simulink model "proj_sim"  (R2024b)
settings: Solver=VariableStepAuto  StartTime=0.0  StopTime=inf  RelTol=1e-3
values from neighbouring files (symbols this model uses):
  gravitation = 9.82    [load_vars.m]
  Weight = scaler * (380 + 72.2)    (= 50.01332)    [load_vars.m]
undefined symbols (not defined in the file or in its folder): battery_voltage, current_limiting_resistor, max_current, Weight_of_tt
libraries: fl_lib x16, nesl_utility x9, sdl_lib x3, ee_lib x1, slpidlib x1, simulink_extras x1, simulink x1
(part 2 of 2)

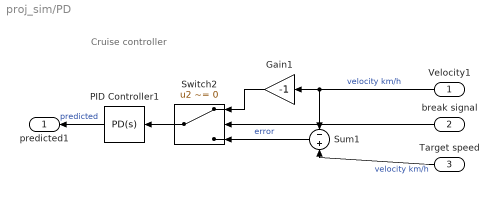
== system proj_sim/PD ==
  note: Cruise controller
  Velocity1 : Inport
  break signal : Inport  Port=2
  Target speed : Inport  Port=3
  Gain1 : Gain  Gain=-1
  PID Controller1 : slpidlib/PID Controller  Controller=PD  Form=Parallel  TimeDomain=Continuous-time  UseExternalTs=off  SampleTime=-1  IntegratorMethod=Forward Euler  FilterMethod=Forward Euler  ControllerParametersSource=internal  P=.5  I=0.0049382534879437  UseKiTs=off  D=.5  UseExternalDerivativeSource=off  N=0.174193742009391  UseFilter=on  TunerSelectOption=Transfer Function Based (PID Tuner App)  InitialConditionSource=internal  InitialConditionForIntegrator=0  InitialConditionForFilter=0  DifferentiatorICPrevScaledInput=0  ExternalReset=none  TrackingMode=off  Kt=1  LimitOutput=off  SatLimitsSource=internal  UpperSaturationLimit=inf  LowerSaturationLimit=-inf  LinearizeAsGain=on  AntiWindupMode=none  Kb=1  LimitIntegrator=off  UpperIntegratorSaturationLimit=inf  LowerIntegratorSaturationLimit=-inf  POutMin=[]  POutMax=[]  IOutMin=[]  IOutMax=[]  DOutMin=[]  DOutMax=[]  NOutMin=[]  NOutMax=[]  SumOutMin=[]  SumOutMax=[]  SaturationOutMin=[]  SaturationOutMax=[]  PParamMin=[]  PParamMax=[]  IParamMin=[]  IParamMax=[]  DParamMin=[]  DParamMax=[]  NParamMin=[]  NParamMax=[]  KbParamMin=[]  KbParamMax=[]  KtParamMin=[]  KtParamMax=[]  KbOutMin=[]  KbOutMax=[]  KtOutMin=[]  KtOutMax=[]  IntegratorOutMin=[]  IntegratorOutMax=[]  FilterOutMin=[]  FilterOutMax=[]  SumI1OutMin=[]  SumI1OutMax=[]  SumI2OutMin=[]  SumI2OutMax=[]  SumI3OutMin=[]  SumI3OutMax=[]  SumI4OutMin=[]  SumI4OutMax=[]  SumDOutMin=[]  SumDOutMax=[]  DifferentiatorOutMin=[]  DifferentiatorOutMax=[]  FilterDiffOutCoefMin=[]  FilterDiffOutCoefMax=[]  ReciprocalOutMin=[]  ReciprocalOutMax=[]  SumDenOutMin=[]  SumDenOutMax=[]  SumNumOutMin=[]  SumNumOutMax=[]  DivideOutMin=[]  DivideOutMax=[]  UdiffTsProdOutMin=[]  UdiffTsProdOutMax=[]  NTsProdOutMin=[]  NTsProdOutMax=[]  UintegralTsProdOutMin=[]  UintegralTsProdOutMax=[]  UngainTsProdOutMin=[]  UngainTsProdOutMax=[]  ClampingZeroOutDataTypeStr=Inherit: Inherit via back propagation  ClampingZeroOutMin=[]  ClampingZeroOutMax=[]  FilterDenConstantOutDataTypeStr=Inherit: Inherit via back propagation  FilterDenConstantOutMin=[]  FilterDenConstantOutMax=[]  PCopyOutDataTypeStr=Inherit: Inherit via back propagation  PCopyOutMin=[]  PCopyOutMax=[]  NCopyOutDataTypeStr=Inherit: Inherit via back propagation  NCopyOutMin=[]  NCopyOutMax=[]  IntegratorContinuousStateAttributes=''  IntegratorStateMustResolveToSignalObject=off  IntegratorRTWStateStorageClass=Auto  FilterContinuousStateAttributes=''  FilterStateMustResolveToSignalObject=off  FilterRTWStateStorageClass=Auto  ParallelPVariant=InternalParameters  IdealPVariant=Disabled  IVariant=Disabled  DVariant=InternalParameters  IntegratorVariant=Disabled  SatVariant=Disabled  AWVariant=Disabled  PCopyVariant=Disabled  TRVariant=Disabled  FdbkBlocksVariant=Forward  IdealPFdbkVariant=Disabled  SatFdbkVariant=Disabled  DerivativeFilterVariant=ContFilter  NVariant=InternalParameters  NCopyVariant=Disabled  FilterICVariant=InternalICsFilter  IntegratorICVariant=Disabled  ExternalResetVariant=Disabled  TRSumVariant=Passthrough  SumFdbkVariant=Disabled  SumVariant=Sum_PD  TsampFilterVariant=InternalTs  TsampNgainVariant=Passthrough  TsampIntegralVariant=Disabled_SignalSpec  ExternalSaturationOutDataTypeStr=Inherit: Same as second input  DerivativeSourceVariant=ErrorSignal  PreIntVariant=InternalPreInt
  Sum1 : Sum  Inputs=-+
  Switch2 : Switch  Criteria=u2 ~= 0  SaturateOnIntegerOverflow=off  InputSameDT=off
  predicted1 : Outport
  wires:
  Gain1/1 -> Switch2/1
  Velocity1/1 -> Sum1/1, Gain1/1  "velocity km/h"
  Sum1/1 -> Switch2/3  "error"
  Switch2/1 -> PID Controller1/1
  break signal/1 -> Switch2/2
  PID Controller1/1 -> predicted1/1  "predicted"
  Target speed/1 -> Sum1/2  "velocity km/h"

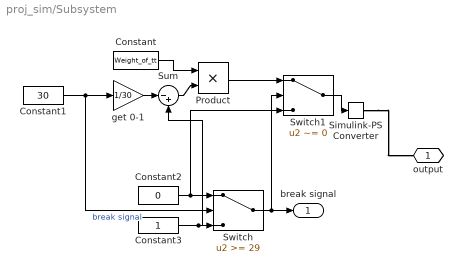
== system proj_sim/Subsystem ==
  Constant : Constant  Value=Weight_of_tt
  Constant1 : Constant  Value=30
  Constant2 : Constant  Value=0
  Constant3 : Constant
  Product : Product
  Simulink-PS Converter : nesl_utility/Simulink-PS Converter  PhysicalDomain=network_engine_domain  SubClassName=ps_input  LeftPortType=input  RightPortType=output  PseudoPeriodic=off  Frequencies=[]  NoiseDistribution=none  NoiseParameters=[]  Unit=1  AffineConversion=off  FilteringAndDerivatives=provide  SimscapeFilterOrder=1  InputFilterTimeConstant=0.001  UdotUserProvided=0
  Sum : Sum  Inputs=|-+
  Switch : Switch  Threshold=29  SaturateOnIntegerOverflow=off  InputSameDT=off
  Switch1 : Switch  Criteria=u2 ~= 0  Threshold=30  SaturateOnIntegerOverflow=off  InputSameDT=off
  get 0-1 : Gain  Gain=1/30
  output : PMIOPort  Side=Right
  break signal : Outport
  wires:
  Constant2/1 -> Switch/1, Switch1/3
  Constant1/1 -> get 0-1/1, Switch/2  "break signal"
  Switch1/1 -> Simulink-PS Converter/1
  Switch/1 -> Switch1/2, break signal/1
  Constant3/1 -> Sum/2, Switch/3
  Constant/1 -> Product/1
  Product/1 -> Switch1/1
  get 0-1/1 -> Sum/1
  Sum/1 -> Product/2
  connections:
  Simulink-PS Converter/RConn1 -- output/RConn1

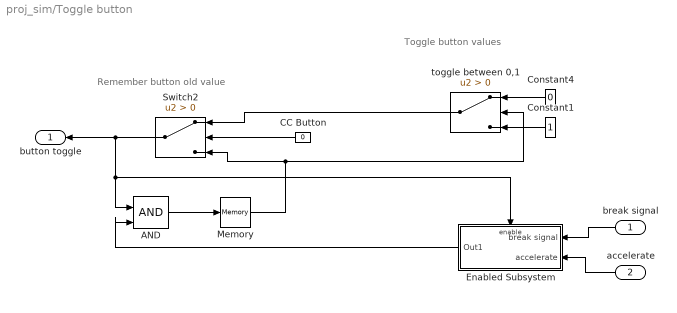
== system proj_sim/Toggle button ==
  note: Toggle button values
  note: Remember button old value
  break signal : Inport
  accelerate : Inport  Port=2
  AND : Logic  IconShape=distinctive  AllPortsSameDT=off  OutDataTypeStr=boolean
  CC Button : Constant  Value=0
  Constant1 : Constant
  Constant4 : Constant  Value=0
  Enabled Subsystem : Subsystem  TreatAsAtomicUnit=on
  Memory : Memory
  Switch2 : Switch  Criteria=u2 > Threshold  SaturateOnIntegerOverflow=off  InputSameDT=off
  toggle between 0,1 : Switch  Criteria=u2 > Threshold  SaturateOnIntegerOverflow=off  InputSameDT=off
  button toggle : Outport
  wires:
  Memory/1 -> toggle between 0,1/2, Switch2/3
  Constant4/1 -> toggle between 0,1/1
  Constant1/1 -> toggle between 0,1/3
  CC Button/1 -> Switch2/2
  toggle between 0,1/1 -> Switch2/1
  break signal/1 -> Enabled Subsystem/1(break signal)
  accelerate/1 -> Enabled Subsystem/2(accelerate)
  AND/1 -> Memory/1
  Switch2/1 -> Enabled Subsystem/Enable, AND/1, button toggle/1
  Enabled Subsystem/1(Out1) -> AND/2

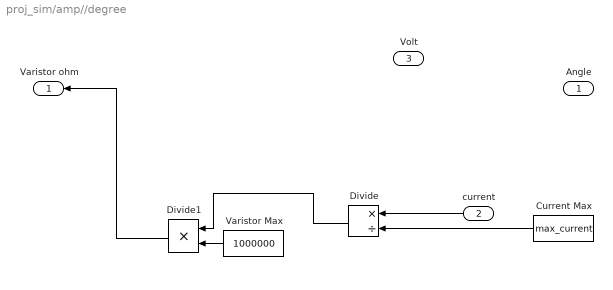
== system proj_sim/amp//degree ==
  Angle : Inport
  current : Inport  Port=2
  Volt : Inport  Port=3
  Current Max : Constant  Value=max_current
  Divide : Product  Inputs=*/
  Divide1 : Product  Inputs=**
  Varistor Max : Constant  Value=1000000
  Varistor ohm : Outport
  wires:
  current/1 -> Divide/1
  Current Max/1 -> Divide/2
  Divide1/1 -> Varistor ohm/1
  Varistor Max/1 -> Divide1/2
  Divide/1 -> Divide1/1

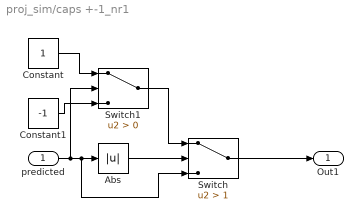
== system proj_sim/caps +-1_nr1 ==
  predicted : Inport
  Abs : Abs  SaturateOnIntegerOverflow=off
  Constant : Constant
  Constant1 : Constant  Value=-1
  Switch : Switch  Criteria=u2 > Threshold  Threshold=1  SaturateOnIntegerOverflow=off  InputSameDT=off
  Switch1 : Switch  Criteria=u2 > Threshold  SaturateOnIntegerOverflow=off  InputSameDT=off
  Out1 : Outport
  wires:
  predicted/1 -> Switch1/2, Switch/3, Abs/1
  Abs/1 -> Switch/2
  Constant/1 -> Switch1/1
  Constant1/1 -> Switch1/3
  Switch1/1 -> Switch/1
  Switch/1 -> Out1/1

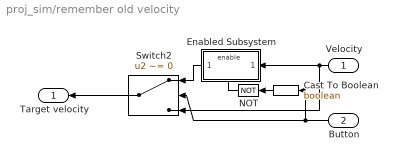
== system proj_sim/remember old velocity ==
  Velocity : Inport
  Button : Inport  Port=2
  Cast To Boolean : DataTypeConversion  OutDataTypeStr=boolean  SaturateOnIntegerOverflow=off  RndMeth=Floor
  Enabled Subsystem : Subsystem  TreatAsAtomicUnit=on
  NOT : Logic  Operator=NOT  IconShape=distinctive  AllPortsSameDT=off  OutDataTypeStr=boolean
  Switch2 : Switch  Criteria=u2 ~= 0  SaturateOnIntegerOverflow=off  InputSameDT=off
  Target velocity : Outport
  wires:
  Switch2/1 -> Target velocity/1
  Velocity/1 -> Enabled Subsystem/1(Velocity), Switch2/3
  Button/1 -> Cast To Boolean/1, Switch2/2
  NOT/1 -> Enabled Subsystem/Enable
  Enabled Subsystem/1(Out1) -> Switch2/1
  Cast To Boolean/1 -> NOT/1

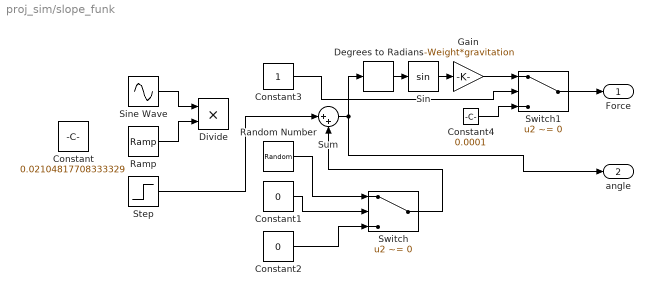
== system proj_sim/slope_funk ==
  Constant : Constant  Value=0.02104817708333329
  Constant1 : Constant  Value=0
  Constant2 : Constant  Value=0
  Constant3 : Constant
  Constant4 : Constant  Value=0.0001
  Degrees to Radians : simulink_extras/Transformations/Degrees to Radians
  Divide : Product  Inputs=**
  Gain : Gain  Gain=-Weight*gravitation
  Ramp : simulink/Sources/Ramp  slope=0.001  start=600  InitialOutput=0
  Random Number : RandomNumber  SampleTime=0.01
  Sin : Trigonometry
  Sine Wave : Sin  Frequency=0.01  SampleTime=0
  Step : Step  Time=600  After=0  SampleTime=0
  Sum : Sum  Inputs=|++
  Switch : Switch  Criteria=u2 ~= 0  SaturateOnIntegerOverflow=off  InputSameDT=off
  Switch1 : Switch  Criteria=u2 ~= 0  SaturateOnIntegerOverflow=off  InputSameDT=off
  Force : Outport
  angle : Outport  Port=2
  wires:
  Degrees to Radians/1 -> Sin/1
  Sin/1 -> Gain/1
  Random Number/1 -> Switch/1
  Constant1/1 -> Switch/2
  Constant2/1 -> Switch/3
  Switch/1 -> Sum/2
  Sum/1 -> angle/1, Degrees to Radians/1
  Constant3/1 -> Switch1/2
  Constant4/1 -> Switch1/3
  Gain/1 -> Switch1/1
  Switch1/1 -> Force/1
  Sine Wave/1 -> Divide/1
  Ramp/1 -> Divide/2
  Step/1 -> Sum/1

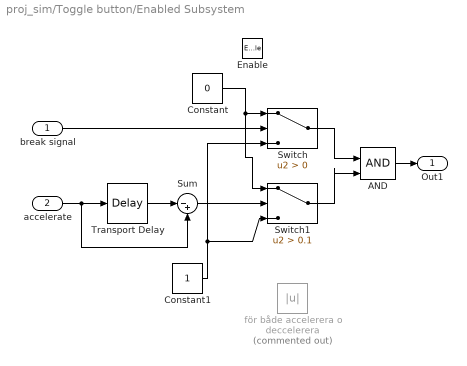
== system proj_sim/Toggle button/Enabled Subsystem ==
  break signal : Inport
  accelerate : Inport  Port=2
  Enable : EnablePort
  AND : Logic  IconShape=distinctive  AllPortsSameDT=off  OutDataTypeStr=boolean
  Constant : Constant  Value=0
  Constant1 : Constant
  Sum : Sum  Inputs=|-+
  Switch : Switch  Criteria=u2 > Threshold  SaturateOnIntegerOverflow=off  InputSameDT=off
  Switch1 : Switch  Criteria=u2 > Threshold  Threshold=0.1  SaturateOnIntegerOverflow=off  InputSameDT=off
  Transport Delay : TransportDelay
  för både accelerera o deccelerera : Abs  Commented=on  SaturateOnIntegerOverflow=off
  Out1 : Outport  InitialOutput=1
  wires:
  break signal/1 -> Switch/2
  Transport Delay/1 -> Sum/1
  Sum/1 -> Switch1/2
  accelerate/1 -> Sum/2, Transport Delay/1
  Constant/1 -> Switch1/1, Switch/1
  Constant1/1 -> Switch1/3, Switch/3
  AND/1 -> Out1/1
  Switch/1 -> AND/1
  Switch1/1 -> AND/2

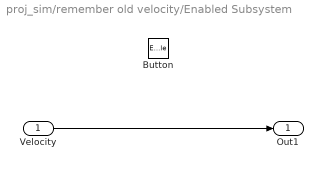
== system proj_sim/remember old velocity/Enabled Subsystem ==
  Velocity : Inport
  Button : EnablePort
  Out1 : Outport
  wires:
  Velocity/1 -> Out1/1
